simulink model "ControladoresPAMH"  (R2024b)
settings: Solver=VariableStepAuto  StartTime=0.0  StopTime=20.0  RelTol=1e-3
model workspace (MATLAB code in the model file):
  | Gn = 5.3881;
  | Gd = [1 0.2673 15.33];
values from neighbouring files (symbols this model uses):
  A = modelmat.a'    [PAMH_Control.m]    (also in pamhws.mat = [0  1; -15.3273076885  -0.267288862263])
  B = modelmat.c'    [PAMH_Control.m]    (also in pamhws.mat = [0 5.38807940163])
  C = modelmat.b'    [PAMH_Control.m]    (also in pamhws.mat = [1 0])
  den_pid = [1 1.6 0]    [pamhws.mat]
  den_pidimc = [1 1.37931034483 0]    [pamhws.mat]
  K = Ks(:,1:2)    [PAMH_Control.m]    (also in pamhws.mat = [-1.40213369651 1.00828342212])
  K_q = Kq(:,1:2)    [PAMH_Control.m]    (also in pamhws.mat = [3.77422787432 3.3272869412])
  KI = -Ks(:,3:3)    [PAMH_Control.m]    (also in pamhws.mat = 0.721964119315)
  KI_q = -Kq(:,3:3)    [PAMH_Control.m]    (also in pamhws.mat = 3.80788655293)
  Kq = lqr(As,Bs,Qs,Rs)    [PAMH_Control.m]    (also in pamhws.mat = [3.77422787432 3.3272869412 -3.80788655293])
  Ks = acker(As,Bs,P)    [PAMH_Control.m]    (also in pamhws.mat = [-1.40213369651 1.00828342212 -0.721964119315])
  num_pid = [0.159054768799 0.042499434223 2.43784361497]    [pamhws.mat]
  num_pidimc = [0.0882734312885 0.0235945050171 1.35299404208]    [pamhws.mat]
undefined symbols (not defined in the file or in its folder): den_pidt, num_pidt
libraries: slpidlib x2
settings Model: Creator=nagel  LastModifiedBy=wilbe

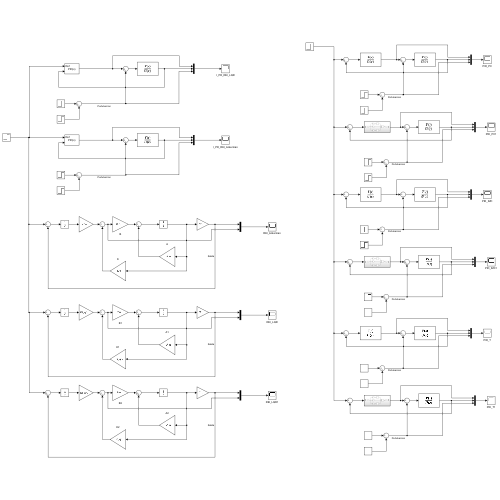
[thumbnail: Simulink's stored preview of the top-level diagram]
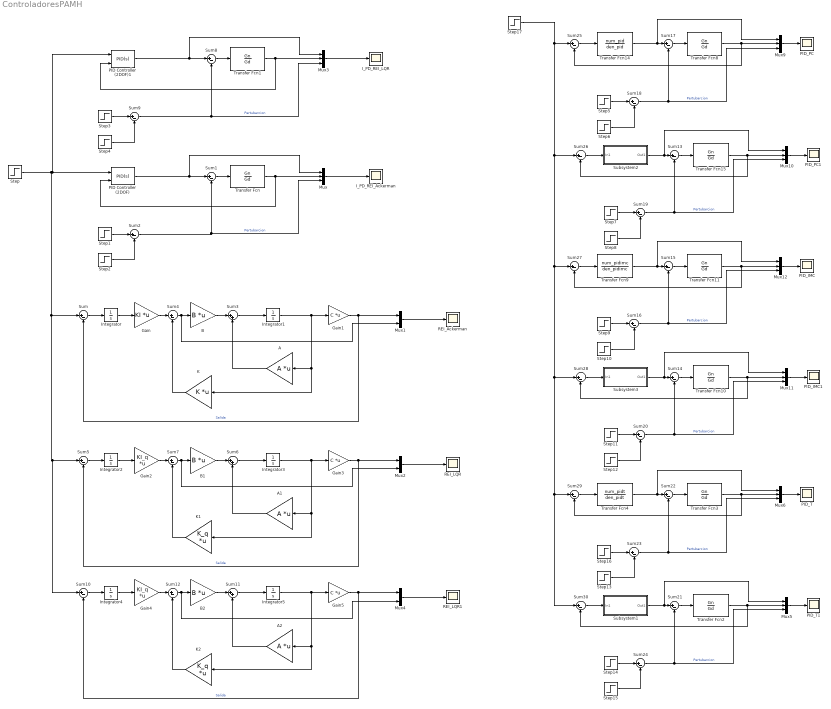
== system ControladoresPAMH ==
  A : Gain  Gain=A  Multiplication=Matrix(K*u)
  A1 : Gain  Gain=A  Multiplication=Matrix(K*u)
  A2 : Gain  Gain=A  Multiplication=Matrix(K*u)
  B : Gain  Gain=B  Multiplication=Matrix(K*u)
  B1 : Gain  Gain=B  Multiplication=Matrix(K*u)
  B2 : Gain  Gain=B  Multiplication=Matrix(K*u)
  Gain : Gain  Gain=KI  Multiplication=Matrix(K*u)
  Gain1 : Gain  Gain=C  Multiplication=Matrix(K*u)
  Gain2 : Gain  Gain=KI_q  Multiplication=Matrix(K*u)
  Gain3 : Gain  Gain=C  Multiplication=Matrix(K*u)
  Gain4 : Gain  Gain=KI_q  Multiplication=Matrix(K*u)
  Gain5 : Gain  Gain=C  Multiplication=Matrix(K*u)
  I_PD_REI_Ackerman : Scope
  I_PD_REI_LQR : Scope
  Integrator{,1..5} (6 alike) : Integrator
  K : Gain  Gain=K  Multiplication=Matrix(K*u)
  K1 : Gain  Gain=K_q  Multiplication=Matrix(K*u)
  K2 : Gain  Gain=K_q  Multiplication=Matrix(K*u)
  Mux{,3,5..6,9..12} (8 alike) : Mux  Inputs=3
  Mux1 : Mux  Inputs=2
  Mux2 : Mux  Inputs=2
  Mux4 : Mux  Inputs=2
  PID Controller (2DOF) : slpidlib/PID Controller (2DOF)  Controller=PID  Form=Parallel  TimeDomain=Continuous-time  UseExternalTs=off  SampleTime=-1  IntegratorMethod=Forward Euler  FilterMethod=Forward Euler  ControllerParametersSource=internal  P=Ks(1)  I=-Ks(3)  UseKiTs=off  D=Ks(2)  UseExternalDerivativeSource=off  N=5  UseFilter=on  b=0  c=0  TunerSelectOption=Transfer Function Based (PID Tuner App)  InitialConditionSource=internal  InitialConditionForIntegrator=0  InitialConditionForFilter=0  DifferentiatorICPrevScaledInput=0  ExternalReset=none  TrackingMode=off  Kt=1  LimitOutput=off  SatLimitsSource=internal  UpperSaturationLimit=inf  LowerSaturationLimit=-inf  LinearizeAsGain=on  AntiWindupMode=none  Kb=1  LimitIntegrator=off  UpperIntegratorSaturationLimit=inf  LowerIntegratorSaturationLimit=-inf  POutMin=[]  POutMax=[]  IOutMin=[]  IOutMax=[]  DOutMin=[]  DOutMax=[]  NOutMin=[]  NOutMax=[]  bOutMin=[]  bOutMax=[]  cOutMin=[]  cOutMax=[]  SumOutMin=[]  SumOutMax=[]  SaturationOutMin=[]  SaturationOutMax=[]  PParamMin=[]  PParamMax=[]  IParamMin=[]  IParamMax=[]  DParamMin=[]  DParamMax=[]  NParamMin=[]  NParamMax=[]  bParamMin=[]  bParamMax=[]  cParamMin=[]  cParamMax=[]  KbParamMin=[]  KbParamMax=[]  KtParamMin=[]  KtParamMax=[]  KbOutMin=[]  KbOutMax=[]  KtOutMin=[]  KtOutMax=[]  IntegratorOutMin=[]  IntegratorOutMax=[]  FilterOutMin=[]  FilterOutMax=[]  SumI1OutMin=[]  SumI1OutMax=[]  SumI2OutMin=[]  SumI2OutMax=[]  SumI3OutMin=[]  SumI3OutMax=[]  SumI4OutMin=[]  SumI4OutMax=[]  SumDOutMin=[]  SumDOutMax=[]  Sum1OutMin=[]  Sum1OutMax=[]  Sum2OutMin=[]  Sum2OutMax=[]  Sum3OutMin=[]  Sum3OutMax=[]  DifferentiatorOutMin=[]  DifferentiatorOutMax=[]  FilterDiffOutCoefMin=[]  FilterDiffOutCoefMax=[]  ReciprocalOutMin=[]  ReciprocalOutMax=[]  SumDenOutMin=[]  SumDenOutMax=[]  SumNumOutMin=[]  SumNumOutMax=[]  DivideOutMin=[]  DivideOutMax=[]  UdiffTsProdOutMin=[]  UdiffTsProdOutMax=[]  NTsProdOutMin=[]  NTsProdOutMax=[]  UintegralTsProdOutMin=[]  UintegralTsProdOutMax=[]  UngainTsProdOutMin=[]  UngainTsProdOutMax=[]  ClampingZeroOutDataTypeStr=Inherit: Inherit via back propagation  ClampingZeroOutMin=[]  ClampingZeroOutMax=[]  FilterDenConstantOutDataTypeStr=Inherit: Inherit via back propagation  FilterDenConstantOutMin=[]  FilterDenConstantOutMax=[]  PCopyOutDataTypeStr=Inherit: Inherit via back propagation  PCopyOutMin=[]  PCopyOutMax=[]  NCopyOutDataTypeStr=Inherit: Inherit via back propagation  NCopyOutMin=[]  NCopyOutMax=[]  IntegratorContinuousStateAttributes=''  IntegratorStateMustResolveToSignalObject=off  IntegratorRTWStateStorageClass=Auto  FilterContinuousStateAttributes=''  FilterStateMustResolveToSignalObject=off  FilterRTWStateStorageClass=Auto  ParallelPVariant=InternalParameters  IdealPVariant=Disabled  IVariant=InternalParameters  DVariant=InternalParameters  bVariant=InternalParameters  cVariant=InternalParameters  IntegratorVariant=Continuous  SatVariant=Disabled  AWVariant=Passthrough  PCopyVariant=Disabled  TRVariant=Disabled  FdbkBlocksVariant=Forward  IdealPFdbkVariant=Disabled  SatFdbkVariant=Disabled  DerivativeFilterVariant=ContFilter  NVariant=InternalParameters  NCopyVariant=Disabled  FilterICVariant=InternalICsFilter  IntegratorICVariant=InternalICs  ExternalResetVariant=Disabled  TRSumVariant=Passthrough  SumFdbkVariant=Disabled  SumVariant=Sum_PID  TsampFilterVariant=InternalTs  TsampNgainVariant=Passthrough  TsampIntegralVariant=Disabled_SignalSpec  ExternalSaturationOutDataTypeStr=Inherit: Same as second input  DerivativeSourceVariant=ErrorSignal  PreIntVariant=InternalPreInt
  PID Controller (2DOF)1 : slpidlib/PID Controller (2DOF)  Controller=PID  Form=Parallel  TimeDomain=Continuous-time  UseExternalTs=off  SampleTime=-1  IntegratorMethod=Forward Euler  FilterMethod=Forward Euler  ControllerParametersSource=internal  P=Kq(1)  I=-Kq(3)  UseKiTs=off  D=Kq(2)  UseExternalDerivativeSource=off  N=5  UseFilter=on  b=0  c=0  TunerSelectOption=Transfer Function Based (PID Tuner App)  InitialConditionSource=internal  InitialConditionForIntegrator=0  InitialConditionForFilter=0  DifferentiatorICPrevScaledInput=0  ExternalReset=none  TrackingMode=off  Kt=1  LimitOutput=off  SatLimitsSource=internal  UpperSaturationLimit=inf  LowerSaturationLimit=-inf  LinearizeAsGain=on  AntiWindupMode=none  Kb=1  LimitIntegrator=off  UpperIntegratorSaturationLimit=inf  LowerIntegratorSaturationLimit=-inf  POutMin=[]  POutMax=[]  IOutMin=[]  IOutMax=[]  DOutMin=[]  DOutMax=[]  NOutMin=[]  NOutMax=[]  bOutMin=[]  bOutMax=[]  cOutMin=[]  cOutMax=[]  SumOutMin=[]  SumOutMax=[]  SaturationOutMin=[]  SaturationOutMax=[]  PParamMin=[]  PParamMax=[]  IParamMin=[]  IParamMax=[]  DParamMin=[]  DParamMax=[]  NParamMin=[]  NParamMax=[]  bParamMin=[]  bParamMax=[]  cParamMin=[]  cParamMax=[]  KbParamMin=[]  KbParamMax=[]  KtParamMin=[]  KtParamMax=[]  KbOutMin=[]  KbOutMax=[]  KtOutMin=[]  KtOutMax=[]  IntegratorOutMin=[]  IntegratorOutMax=[]  FilterOutMin=[]  FilterOutMax=[]  SumI1OutMin=[]  SumI1OutMax=[]  SumI2OutMin=[]  SumI2OutMax=[]  SumI3OutMin=[]  SumI3OutMax=[]  SumI4OutMin=[]  SumI4OutMax=[]  SumDOutMin=[]  SumDOutMax=[]  Sum1OutMin=[]  Sum1OutMax=[]  Sum2OutMin=[]  Sum2OutMax=[]  Sum3OutMin=[]  Sum3OutMax=[]  DifferentiatorOutMin=[]  DifferentiatorOutMax=[]  FilterDiffOutCoefMin=[]  FilterDiffOutCoefMax=[]  ReciprocalOutMin=[]  ReciprocalOutMax=[]  SumDenOutMin=[]  SumDenOutMax=[]  SumNumOutMin=[]  SumNumOutMax=[]  DivideOutMin=[]  DivideOutMax=[]  UdiffTsProdOutMin=[]  UdiffTsProdOutMax=[]  NTsProdOutMin=[]  NTsProdOutMax=[]  UintegralTsProdOutMin=[]  UintegralTsProdOutMax=[]  UngainTsProdOutMin=[]  UngainTsProdOutMax=[]  ClampingZeroOutDataTypeStr=Inherit: Inherit via back propagation  ClampingZeroOutMin=[]  ClampingZeroOutMax=[]  FilterDenConstantOutDataTypeStr=Inherit: Inherit via back propagation  FilterDenConstantOutMin=[]  FilterDenConstantOutMax=[]  PCopyOutDataTypeStr=Inherit: Inherit via back propagation  PCopyOutMin=[]  PCopyOutMax=[]  NCopyOutDataTypeStr=Inherit: Inherit via back propagation  NCopyOutMin=[]  NCopyOutMax=[]  IntegratorContinuousStateAttributes=''  IntegratorStateMustResolveToSignalObject=off  IntegratorRTWStateStorageClass=Auto  FilterContinuousStateAttributes=''  FilterStateMustResolveToSignalObject=off  FilterRTWStateStorageClass=Auto  ParallelPVariant=InternalParameters  IdealPVariant=Disabled  IVariant=InternalParameters  DVariant=InternalParameters  bVariant=InternalParameters  cVariant=InternalParameters  IntegratorVariant=Continuous  SatVariant=Disabled  AWVariant=Passthrough  PCopyVariant=Disabled  TRVariant=Disabled  FdbkBlocksVariant=Forward  IdealPFdbkVariant=Disabled  SatFdbkVariant=Disabled  DerivativeFilterVariant=ContFilter  NVariant=InternalParameters  NCopyVariant=Disabled  FilterICVariant=InternalICsFilter  IntegratorICVariant=InternalICs  ExternalResetVariant=Disabled  TRSumVariant=Passthrough  SumFdbkVariant=Disabled  SumVariant=Sum_PID  TsampFilterVariant=InternalTs  TsampNgainVariant=Passthrough  TsampIntegralVariant=Disabled_SignalSpec  ExternalSaturationOutDataTypeStr=Inherit: Same as second input  DerivativeSourceVariant=ErrorSignal  PreIntVariant=InternalPreInt
  PID_IMC : Scope
  PID_IMC1 : Scope
  PID_PC : Scope
  PID_PC1 : Scope
  PID_T : Scope
  PID_T1 : Scope
  REI_Ackerman : Scope
  REI_LQR : Scope
  REI_LQR1 : Scope
  Step : Step  Time=0  After=0.6  SampleTime=0
  Step{1,3,5,7,9,11,14,16} (8 alike) : Step  Time=8  After=0.1  SampleTime=0
  Step{2,4,6,8,10,12..13,15} (8 alike) : Step  Time=14  After=0.1  SampleTime=0
  Step17 : Step  Time=0  After=0.6  SampleTime=0
  Subsystem1 : Subsystem
  Subsystem2 : Subsystem
  Subsystem3 : Subsystem
  Sum{,1..2,4..5,7..10,12..30} (28 alike) : Sum  Inputs=|+-
  Sum11 : Sum  Inputs=|++
  Sum3 : Sum  Inputs=|++
  Sum6 : Sum  Inputs=|++
  Transfer Fcn{,1..3,8,10..11,15} (8 alike) : TransferFcn  Numerator=Gn  Denominator=Gd
  Transfer Fcn14 : TransferFcn  Numerator=num_pid  Denominator=den_pid
  Transfer Fcn4 : TransferFcn  Numerator=num_pidt  Denominator=den_pidt
  Transfer Fcn9 : TransferFcn  Numerator=num_pidimc  Denominator=den_pidimc
  wires:
  Sum1/1 -> Transfer Fcn/1
  Step1/1 -> Sum2/1
  Step2/1 -> Sum2/2
  Sum2/1 -> Mux/3, Sum1/2  "Pertubarcion"
  Transfer Fcn/1 -> PID Controller (2DOF)/2, Mux/2
  PID Controller (2DOF)/1 -> Mux/1, Sum1/1
  Mux/1 -> I_PD_REI_Ackerman/1
  Integrator/1 -> Gain/1
  Sum/1 -> Integrator/1
  Sum3/1 -> Integrator1/1
  A/1 -> Sum3/2
  B/1 -> Sum3/1
  Integrator1/1 -> K/1, A/1, Gain1/1
  Gain/1 -> Sum4/1
  Sum4/1 -> Mux1/2, B/1
  Gain1/1 -> Mux1/1, Sum/2  "Salida"
  K/1 -> Sum4/2
  Mux1/1 -> REI_Ackerman/1
  Integrator3/1 -> K1/1, A1/1, Gain3/1
  Sum7/1 -> Mux2/2, B1/1
  Gain3/1 -> Mux2/1, Sum5/2  "Salida"
  K1/1 -> Sum7/2
  Sum5/1 -> Integrator2/1
  B1/1 -> Sum6/1
  Mux2/1 -> REI_LQR/1
  Sum6/1 -> Integrator3/1
  A1/1 -> Sum6/2
  Gain2/1 -> Sum7/1
  Integrator2/1 -> Gain2/1
  Sum9/1 -> Mux3/3, Sum8/2  "Pertubarcion"
  Sum8/1 -> Transfer Fcn1/1
  Mux3/1 -> I_PD_REI_LQR/1
  Step3/1 -> Sum9/1
  Transfer Fcn1/1 -> PID Controller (2DOF)1/2, Mux3/2
  PID Controller (2DOF)1/1 -> Mux3/1, Sum8/1
  Step4/1 -> Sum9/2
  Integrator4/1 -> Gain4/1
  Sum12/1 -> Mux4/2, B2/1
  Gain4/1 -> Sum12/1
  Gain5/1 -> Mux4/1, Sum10/2  "Salida"
  Sum11/1 -> Integrator5/1
  A2/1 -> Sum11/2
  Sum10/1 -> Integrator4/1
  Integrator5/1 -> K2/1, A2/1, Gain5/1
  K2/1 -> Sum12/2
  B2/1 -> Sum11/1
  Mux4/1 -> REI_LQR1/1
  Transfer Fcn14/1 -> Mux9/1, Sum17/1
  Sum17/1 -> Transfer Fcn8/1
  Mux9/1 -> PID_PC/1
  Sum18/1 -> Mux9/3, Sum17/2  "Pertubarcion"
  Step6/1 -> Sum18/2
  Step5/1 -> Sum18/1
  Step/1 -> Sum10/1, Sum5/1, Sum/1, PID Controller (2DOF)1/1, PID Controller (2DOF)/1
  Transfer Fcn8/1 -> Sum25/2, Mux9/2
  Sum25/1 -> Transfer Fcn14/1
  Sum26/1 -> Subsystem2/1(In1)
  Transfer Fcn15/1 -> Sum26/2, Mux10/2
  Step7/1 -> Sum19/1
  Step8/1 -> Sum19/2
  Mux10/1 -> PID_PC1/1
  Sum13/1 -> Transfer Fcn15/1
  Sum19/1 -> Mux10/3, Sum13/2  "Pertubarcion"
  Subsystem2/1(Out1) -> Mux10/1, Sum13/1
  Sum14/1 -> Transfer Fcn10/1
  Step12/1 -> Sum20/2
  Mux11/1 -> PID_IMC1/1
  Sum20/1 -> Mux11/3, Sum14/2  "Pertubarcion"
  Transfer Fcn10/1 -> Sum28/2, Mux11/2
  Step11/1 -> Sum20/1
  Sum27/1 -> Transfer Fcn9/1
  Transfer Fcn11/1 -> Sum27/2, Mux12/2
  Subsystem3/1(Out1) -> Mux11/1, Sum14/1
  Sum28/1 -> Subsystem3/1(In1)
  Step9/1 -> Sum16/1
  Step10/1 -> Sum16/2
  Mux12/1 -> PID_IMC/1
  Sum15/1 -> Transfer Fcn11/1
  Sum16/1 -> Mux12/3, Sum15/2  "Pertubarcion"
  Transfer Fcn9/1 -> Mux12/1, Sum15/1
  Step17/1 -> Sum25/1, Sum26/1, Sum27/1, Sum29/1, Sum30/1, Sum28/1
  Sum23/1 -> Mux6/3, Sum22/2  "Pertubarcion"
  Mux6/1 -> PID_T/1
  Step16/1 -> Sum23/1
  Sum30/1 -> Subsystem1/1(In1)
  Sum22/1 -> Transfer Fcn3/1
  Subsystem1/1(Out1) -> Mux5/1, Sum21/1
  Transfer Fcn4/1 -> Mux6/1, Sum22/1
  Step13/1 -> Sum23/2
  Transfer Fcn3/1 -> Sum29/2, Mux6/2
  Sum29/1 -> Transfer Fcn4/1
  Step14/1 -> Sum24/1
  Sum24/1 -> Mux5/3, Sum21/2  "Pertubarcion"
  Mux5/1 -> PID_T1/1
  Transfer Fcn2/1 -> Sum30/2, Mux5/2
  Step15/1 -> Sum24/2
  Sum21/1 -> Transfer Fcn2/1

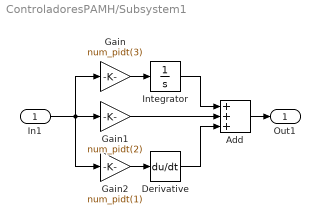
== system ControladoresPAMH/Subsystem1 ==
  In1 : Inport
  Add : Sum  Inputs=+++
  Derivative : Derivative
  Gain : Gain  Gain=num_pidt(3)
  Gain1 : Gain  Gain=num_pidt(2)
  Gain2 : Gain  Gain=num_pidt(1)
  Integrator : Integrator
  Out1 : Outport
  wires:
  In1/1 -> Gain2/1, Gain1/1, Gain/1
  Add/1 -> Out1/1
  Gain/1 -> Integrator/1
  Integrator/1 -> Add/1
  Gain2/1 -> Derivative/1
  Gain1/1 -> Add/2
  Derivative/1 -> Add/3

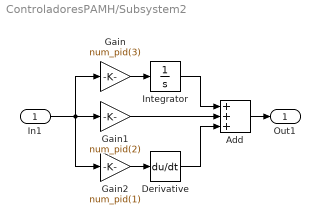
== system ControladoresPAMH/Subsystem2 ==
  In1 : Inport
  Add : Sum  Inputs=+++
  Derivative : Derivative
  Gain : Gain  Gain=num_pid(3)
  Gain1 : Gain  Gain=num_pid(2)
  Gain2 : Gain  Gain=num_pid(1)
  Integrator : Integrator
  Out1 : Outport
  wires:
  In1/1 -> Gain2/1, Gain1/1, Gain/1
  Add/1 -> Out1/1
  Gain/1 -> Integrator/1
  Integrator/1 -> Add/1
  Gain2/1 -> Derivative/1
  Gain1/1 -> Add/2
  Derivative/1 -> Add/3

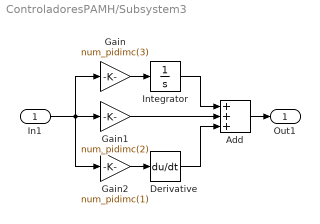
== system ControladoresPAMH/Subsystem3 ==
  In1 : Inport
  Add : Sum  Inputs=+++
  Derivative : Derivative
  Gain : Gain  Gain=num_pidimc(3)
  Gain1 : Gain  Gain=num_pidimc(2)
  Gain2 : Gain  Gain=num_pidimc(1)
  Integrator : Integrator
  Out1 : Outport
  wires:
  In1/1 -> Gain2/1, Gain1/1, Gain/1
  Add/1 -> Out1/1
  Gain/1 -> Integrator/1
  Integrator/1 -> Add/1
  Gain2/1 -> Derivative/1
  Gain1/1 -> Add/2
  Derivative/1 -> Add/3
